simulink model "HEVarchieve"  (R2015a)
settings: Solver=ode45  StartTime=0.0  StopTime=10.0  RelTol=1e-3
undefined symbols (not defined in the file): Hydride, magnitude, Metal, Nickel, Ts
libraries: powerlib x46, driveline x28, simulink_extras x8, electricdrivelib x3, simulink x2, powerlib_extras x2, DC6DriveInternalModels x1
(part 1 of 2)
settings Model: Creator=Elena  LastModifiedBy=Elena

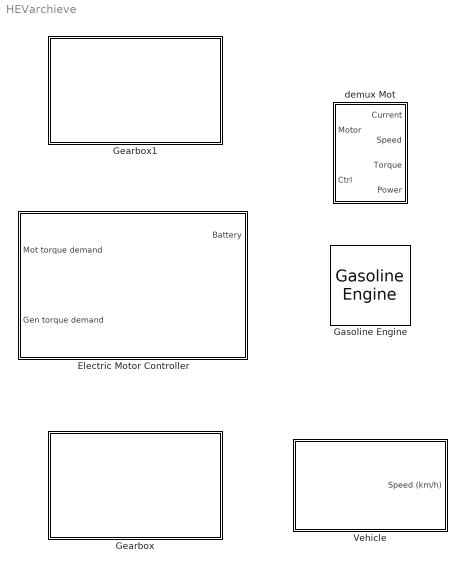
== system HEVarchieve ==
  "Electric Motor Controller " : Subsystem
  Gasoline Engine : driveline/Vehicle Components/Gasoline Engine  power_max=57000  speed_at_power_max=5000  speed_max=6000
      link override Peak torque: LookUpMeth=Interpolation-Extrapolation
  Gearbox : Subsystem
  Gearbox1 : Subsystem
  Vehicle : Subsystem
  demux Mot : Subsystem

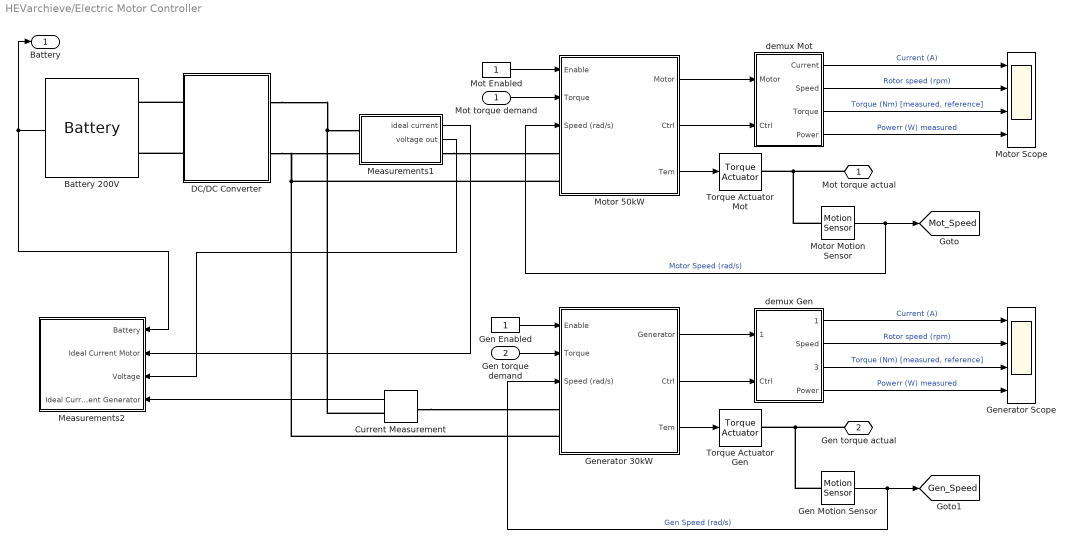
== system HEVarchieve/Electric Motor Controller  ==
  Mot torque demand : Inport
  "Gen torque demand " : Inport  Port=2
  Battery 200V : electricdrivelib/Extra Sources/Battery  BatType=Nickel-Metal-Hydride  ShowDetailedParameters=off  NomV=200  NomQ=6.5  SOC=70  PresetModel=on  MaxQ=7  FullV=235.5932  Dis_rate=1.3  R=0.30769  Normal_OP=6.25  expZone="[216.9492           1.3]"  current=[50 100]  Units=Time  Batt_Tr=30
  Current Measurement : powerlib/Measurements/Current Measurement  PhasorSimulation=off  OutputType=Complex  PSBequivalent=0
  DC/DC Converter : Subsystem
      mask init:
      | [X1,X1m,X2,X2m,X3,X4,Y1,Y1m,Y2,Y2m,Y3,Y4,color1,color2]=spsdrivelogo;
  Gen Enabled : Constant
  Gen Motion Sensor : driveline/Sensors & Actuators/Motion Sensor  Angle=off  x0=0  Velocity=on  Acceleration=off
  Generator 30kW : Subsystem
  Generator Scope : Scope  NumInputPorts=4
      settings: YMin=-5~-5~-5~-5  YMax=5~5~5~5
  Measurements1 : Subsystem
  Measurements2 : Subsystem
  Mot Enabled : Constant
  Motor 50kW : Subsystem
  Motor Motion Sensor : driveline/Sensors & Actuators/Motion Sensor  Angle=off  x0=0  Velocity=on  Acceleration=off
  Motor Scope : Scope  NumInputPorts=4
      settings: YMin=0~0~-100~-5  YMax=250~6000~400~5
  Torque Actuator Gen : driveline/Sensors & Actuators/Torque Actuator
  Torque Actuator Mot : driveline/Sensors & Actuators/Torque Actuator
  demux Gen : Subsystem
  demux Mot : Subsystem
  Mot torque actual : PMIOPort  Port=1  Side=Right
  Gen torque actual : PMIOPort  Port=2  Side=Right
  Battery : Outport
  tag scope: Gen_Speed=global, Mot_Speed=global
  wires:
  Battery 200V/1 -> Measurements2/1(Battery), Battery/1
  Mot Enabled/1 -> Motor 50kW/1(Enable)
  Mot torque demand/1 -> Motor 50kW/2(Torque)
  Motor Motion Sensor/1 -> [Mot_Speed], Motor 50kW/3(Speed (rad/s))  "Motor Speed (rad/s)"
  "Gen torque demand "/1 -> Generator 30kW/2(Torque)
  Gen Enabled/1 -> Generator 30kW/1(Enable)
  Motor 50kW/1(Motor) -> demux Mot/1(Motor)
  Motor 50kW/2(Ctrl) -> demux Mot/2(Ctrl)
  Motor 50kW/3(Tem) -> Torque Actuator Mot/1
  Generator 30kW/3(Tem) -> Torque Actuator Gen/1
  demux Mot/1(Current) -> Motor Scope/1  "Current (A)"
  demux Mot/2(Speed) -> Motor Scope/2  "Rotor speed (rpm)"
  demux Mot/3(Torque) -> Motor Scope/3  "Torque (Nm) [measured, reference]"
  demux Mot/4(Power) -> Motor Scope/4  "Powerr (W) measured"
  Generator 30kW/2(Ctrl) -> demux Gen/2(Ctrl)
  Generator 30kW/1(Generator) -> demux Gen/1(Generator)
  demux Gen/1(Current) -> Generator Scope/1  "Current (A)"
  demux Gen/2(Speed) -> Generator Scope/2  "Rotor speed (rpm)"
  demux Gen/3(Torque) -> Generator Scope/3  "Torque (Nm) [measured, reference]"
  demux Gen/4(Power) -> Generator Scope/4  "Powerr (W) measured"
  Measurements1/2(voltage out) -> Measurements2/3(Voltage)
  Measurements1/1(" ideal current ") -> Measurements2/2(Ideal Current Motor)
  Current Measurement/1 -> Measurements2/4(Ideal Current Generator)
  Gen Motion Sensor/1 -> Generator 30kW/3(Speed (rad/s)), [Gen_Speed]  "Gen Speed (rad/s)"
  connections:
  DC/DC Converter/LConn1 -- Battery 200V/LConn1
  DC/DC Converter/LConn2 -- Battery 200V/LConn2
  Generator 30kW/LConn2 -- Motor 50kW/LConn2 -- Measurements1/LConn2 -- DC/DC Converter/RConn2
  Current Measurement/RConn1 -- DC/DC Converter/RConn1 -- Measurements1/LConn1
  Measurements1/RConn1 -- Motor 50kW/LConn1
  Current Measurement/LConn1 -- Generator 30kW/LConn1
  Gen torque actual/RConn1 -- Torque Actuator Gen/RConn1 -- Gen Motion Sensor/LConn1
  Mot torque actual/RConn1 -- Motor Motion Sensor/LConn1 -- Torque Actuator Mot/RConn1

== system HEVarchieve/Gearbox ==
  Eng Motion Sensor : driveline/Sensors & Actuators/Motion Sensor  Angle=off  x0=0  Velocity=on  Acceleration=off
  Gen Motion Sensor : driveline/Sensors & Actuators/Motion Sensor  Angle=off  x0=0  Velocity=on  Acceleration=off
  Mot Motion Sensor : driveline/Sensors & Actuators/Motion Sensor  Angle=off  x0=0  Velocity=on  Acceleration=off
  Planetary Gear : driveline/Gears/Planetary Gear  Ratio=2.6  Show=off  LinearizationFlag=off  ValidatorFcn=drive_planetarygearblock
  Speed : Scope  NumInputPorts=3
      settings: TimeRange=10  YMin=3.91275~0~37.3  YMax=3.91275~150~37.6  SaveName=ScopeData3  Decimation=10
  T1 : driveline/Sensors & Actuators/Torque Sensor
  Torque Sensor : driveline/Sensors & Actuators/Torque Sensor
  Torque Sensor1 : driveline/Sensors & Actuators/Torque Sensor
  Engine Torque : PMIOPort  Port=1  Side=Left
  Motor Torque : PMIOPort  Port=2  Side=Right
  Generator Torque : PMIOPort  Port=3  Side=Right
  wires:
  Eng Motion Sensor/1 -> Speed/3  "Engine speed (rad/s)"
  Gen Motion Sensor/1 -> Speed/2  "Generator speed (rad/s)"
  Mot Motion Sensor/1 -> Speed/1  "Motor speed (rad/s)"
  connections:
  Torque Sensor/LConn1 -- Planetary Gear/RConn1
  Eng Motion Sensor/LConn1 -- Planetary Gear/LConn1 -- T1/RConn1
  T1/LConn1 -- Engine Torque/RConn1
  Torque Sensor/RConn1 -- Motor Torque/RConn1 -- Mot Motion Sensor/LConn1
  Torque Sensor1/RConn1 -- Gen Motion Sensor/LConn1 -- Generator Torque/RConn1
  Torque Sensor1/LConn1 -- Planetary Gear/RConn2

== system HEVarchieve/Gearbox1 ==
  Eng Motion Sensor : driveline/Sensors & Actuators/Motion Sensor  Angle=off  x0=0  Velocity=on  Acceleration=off
  Gen Motion Sensor : driveline/Sensors & Actuators/Motion Sensor  Angle=off  x0=0  Velocity=on  Acceleration=off
  Mot Motion Sensor : driveline/Sensors & Actuators/Motion Sensor  Angle=off  x0=0  Velocity=on  Acceleration=off
  Planetary Gear : driveline/Gears/Planetary Gear  Ratio=2  Show=off  LinearizationFlag=off  ValidatorFcn=drive_planetarygearblock
  Speed : Scope  NumInputPorts=3
      settings: TimeRange=16  YMin=-100~-20~-200  YMax=500~120~1200  SaveName=ScopeData3  Decimation=10
  Torque Sensor : driveline/Sensors & Actuators/Torque Sensor
  Engine Torque : PMIOPort  Port=1  Side=Left
  Motor Torque : PMIOPort  Port=2  Side=Right
  Generator Torque : PMIOPort  Port=3  Side=Right
  wires:
  Eng Motion Sensor/1 -> Speed/3  "Engine speed (rad/s)"
  Gen Motion Sensor/1 -> Speed/2  "Generator speed (rad/s)"
  Mot Motion Sensor/1 -> Speed/1  "Motor speed (rad/s)"
  connections:
  Planetary Gear/RConn2 -- Gen Motion Sensor/LConn1 -- Generator Torque/RConn1
  Mot Motion Sensor/LConn1 -- Torque Sensor/LConn1 -- Planetary Gear/RConn1 -- Motor Torque/RConn1
  Planetary Gear/LConn1 -- Eng Motion Sensor/LConn1 -- Engine Torque/RConn1

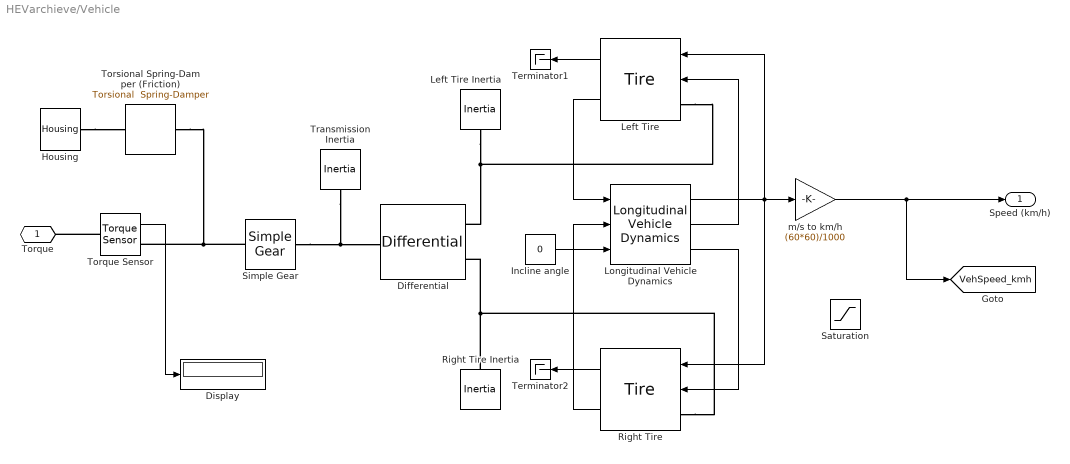
== system HEVarchieve/Vehicle ==
  Differential : driveline/Gears/Differential  R=1  ValidatorFcn=drive_differentialgearblock  SimDrivelineLibraryVersion=1.1
  Display : Display
  Housing : driveline/Solver & Inertias/Housing
  Incline angle : Constant  Value=0
  Left Tire : driveline/Vehicle Components/Tire  r_e=0.3  F_z=3000  F_x_max=3500  kappa_max=10  sigma_k=0.2
  Left Tire Inertia : driveline/Solver & Inertias/Inertia  PortType=p1  BlockClass=Inertia  PhysicalDomain=driveline_domain  I=0.5  Ip=[]  Iv=[]  ShowLeft=off  ShowRight=on
  Longitudinal Vehicle Dynamics : driveline/Vehicle Components/Longitudinal Vehicle Dynamics  m=1325  a=1.35  b=1.35  h=0.5  FA=2.57  C_d=0.26  v0=0
  Right Tire : driveline/Vehicle Components/Tire  r_e=0.3  F_z=3000  F_x_max=3500  kappa_max=10  sigma_k=0.2
  Right Tire Inertia : driveline/Solver & Inertias/Inertia  PortType=p1  BlockClass=Inertia  PhysicalDomain=driveline_domain  I=0.5  Ip=[]  Iv=[]  ShowLeft=off  ShowRight=on
  Saturation : Saturate  UpperLimit=Inf  LowerLimit=0
  Simple Gear : driveline/Gears/Simple Gear  PortType=p1  BlockClass=SimpleGear  PhysicalDomain=driveline_domain  Reversing=off  Ratio=4.113
  Terminator1 : Terminator
  Terminator2 : Terminator
  Torque Sensor : driveline/Sensors & Actuators/Torque Sensor
  Torsional Spring-Damper (Friction) : driveline/Dynamic Elements/Torsional  Spring-Damper  k=0  c=0.1  x0=0  Backlash=0
  Transmission Inertia : driveline/Solver & Inertias/Inertia  PortType=p1  BlockClass=Inertia  PhysicalDomain=driveline_domain  I=0.5  Ip=[]  Iv=[]  ShowLeft=off  ShowRight=on
  m/s to km/h : Gain  Gain=(60*60)/1000
  Torque : PMIOPort  Port=1  Side=Left
  Speed (km/h) : Outport
  tag scope: VehSpeed_kmh=global
  wires:
  Left Tire/2 -> Longitudinal Vehicle Dynamics/1
  Right Tire/2 -> Longitudinal Vehicle Dynamics/2
  Incline angle/1 -> Longitudinal Vehicle Dynamics/3
  Longitudinal Vehicle Dynamics/3 -> Right Tire/2
  Longitudinal Vehicle Dynamics/2 -> Left Tire/2
  Longitudinal Vehicle Dynamics/1 -> m/s to km/h/1, Right Tire/1, Left Tire/1
  Left Tire/1 -> Terminator1/1
  Right Tire/1 -> Terminator2/1
  Torque Sensor/1 -> Display/1
  ? -> Saturation/1
  m/s to km/h/1 -> [VehSpeed_kmh], Speed (km/h)/1
  connections:
  Torque Sensor/LConn1 -- Torque/RConn1
  Torsional Spring-Damper (Friction)/RConn1 -- Simple Gear/LConn1 -- Torque Sensor/RConn1
  Housing/RConn1 -- Torsional Spring-Damper (Friction)/LConn1
  Simple Gear/RConn1 -- Transmission Inertia/RConn1 -- Differential/LConn1
  Left Tire Inertia/RConn1 -- Left Tire/LConn1 -- Differential/RConn1
  Right Tire Inertia/RConn1 -- Right Tire/LConn1 -- Differential/RConn2

== system HEVarchieve/demux Mot ==
  Motor : Inport
  Ctrl : Inport  Port=2
  "+ -> -1" : Gain  Gain=30/pi
  Bus Selector : BusSelector  OutputSignals=Stator current is_a (A),Rotor speed wm (rad/s),Electromagnetic torque Te (N*m)
  Bus Selector1 : BusSelector  OutputSignals=Torque reference (Nm)
  Mux1 : Mux  Inputs=2
  Product : Product  RndMeth=Zero
  Current : Outport
  Speed : Outport  Port=2
  Torque : Outport  Port=3
  Power : Outport  Port=4
  wires:
  "+ -> -1"/1 -> Speed/1
  Motor/1 -> Bus Selector/1
  Ctrl/1 -> Bus Selector1/1
  Bus Selector/2 -> "+ -> -1"/1, Product/2  "<Rotor speed wm (rad/s)>"
  Bus Selector/3 -> Product/1, Mux1/1  "<Electromagnetic torque Te (N*m)>"
  Bus Selector1/1 -> Mux1/2  "<Torque reference (Nm)>"
  Mux1/1 -> Torque/1
  Bus Selector/1 -> Current/1  "<Stator current is_a (A)>"
  Product/1 -> Power/1

== system HEVarchieve/Electric Motor Controller /DC//DC Converter ==
  Bus DC controller : Subsystem
  DC/DC converter : Subsystem
  Ubus Ref : Constant  Value=500
  +VDC : PMIOPort  Tag=PMCPort  Port=1  Side=Right
  -VDC : PMIOPort  Tag=PMCPort  Port=2  Side=Right
  + Bat : PMIOPort  Tag=PMCPort  Port=3  Side=Left
  - Bat : PMIOPort  Tag=PMCPort  Port=4  Side=Left
  wires:
  Ubus Ref/1 -> Bus DC controller/2(Uref)
  Bus DC controller/1(Duty cycle) -> DC/DC converter/1(Duty Cycle)
  DC/DC converter/1(UBus) -> Bus DC controller/1(Ubus)
  connections:
  +VDC/RConn1 -- DC/DC converter/LConn1
  -VDC/RConn1 -- DC/DC converter/LConn2
  + Bat/RConn1 -- DC/DC converter/RConn1
  - Bat/RConn1 -- DC/DC converter/RConn2

== system HEVarchieve/Electric Motor Controller /Generator 30kW ==
  Enable : Inport
  Torque : Inport  Port=2
  Speed (rad/s) : Inport  Port=3
  Bus Selector : BusSelector  OutputSignals=Rotor speed wm (rad/s),Rotor angle thetam (rad),Electromagnetic torque Te (N*m)
  Measures : electricdrivelib/AC drives/PM Synchronous Motor Drive/Measures
  Mux : Subsystem
  PMSM1 : powerlib/Machines/Permanent Magnet Synchronous Machine  NbPhases=3  FluxDistribution=Sinusoidal  RotorType=Salient-pole  MechanicalLoad=Speed w  PresetModel=No  ShowDetailedParameters=on  MeasurementBus=off  Resistance=0.05  Inductance=0  dqInductances=[0.000635 0.000635]  La=0.000835  MachineConstant=Flux linkage established by magnets (V.s)  Flux=0.192  VoltageCst=34.8249  TorqueCst=0.288  Flat=0  Mechanical=[0.011 0.001889/4 4/4]  PolePairs=1  InitialConditions=[0,0, 0,0,0]  InitialConditions5ph=[0 0 0 0 0 0]  TsPowergui=0  TsBlock=-1  RefAngle=90 degrees behind phase A axis (modified Park)
      settings: AttributesFormatString=\n
  Speed Controller : Subsystem  mask(Speed controller){SwK=Torque regulation, bs=1800, ramp=[-5000,5000], kp=(1/5)/4, ki=(50/5)/4/3, fc=(1000/10)/2, ctrl_sat=[-45,45], Tsc=Ts}
      mask prompts: SwK "Regulation type"; bs "Base speed (rpm)"; ramp "Speed reference ramp (rpm/s) [deceleration,acceleration]"; kp "Proportional gain"; ki "Integral gain"; fc "Speed measurement - low-pass filter cutoff frequency (Hz)"; ctrl_sat "Controller output torque saturation (N.m) [negative,positive]"; Tsc "Controller sampling time (s)"
      mask help: This block implements a PI speed regulator.
      mask init:
      | [X1,X1m,X2,X2m,X3,X4,Y1,Y1m,Y2,Y2m,Y3,Y4,color1,color2]=spsdrivelogo;
      mask TypeOptions SwK: Speed regulation | Torque regulation
      mask Display:
      | patch([X1 X1m],[Y1 Y1m],color1);
      | patch(X3,Y3,color2);
      | plot([X1 X1m X2 X2m X3 X4],[Y1 Y1m Y2 Y2m Y3 Y4]);
  Three-phase Inverter : Subsystem  mask(SPSdrives Converter){Arms=3, SnubberResistance=5000, SnubberCapacitance=inf, Device=IGBT / Diodes, Ron=1e-3, Lon=0, ForwardVoltages=[0.8,0.8], ForwardVoltage=0, GTOparameters=[0,0], IGBTparameters=[1e-6,2e-6], Measurements=All voltages and currents, SourceFrequency=60, dqInductances=[0.000635,0.000635], Flux=0.192, Resistance=0.05, p=4/4, converterType=Inverter}
      mask prompts: Arms "Number of bridge arms:"; SnubberResistance "Snubber resistance Rs (Ohms)"; SnubberCapacitance "Snubber capacitance Cs (F)"; Device "Power Electronic device"; Ron "Ron (Ohms)"; Lon "Lon (H)"; ForwardVoltages "Forward voltages  [ Device Vf(V) , Diode Vfd(V)]"; ForwardVoltage "Forward voltage Vf (V)"; GTOparameters "[  Tf (s) , Tt (s)  ]"; IGBTparameters "[  Tf (s) , Tt (s)  ]"; SourceFrequency "Source Frequency (Hz)"; dqInductances "PMSM-Inductances [ Ld(H) Lq(H) ]:"; Flux "PMSM-Flux induced by magnets (Wb):"; Resistance "PMSM-Stator resistance Rs (ohm):"; p "PMSM-Pairs of poles p:"; converterType "Converter type:"
      mask init:
      | Ld=dqInductances(1);
      | Lq=dqInductances(2);
      | Fcs=6*SourceFrequency/10;
      settings: OpenFcn=power_openblockproxy();
      mask Help: web(psbhelp);
      mask TypeOptions Arms: 1 | 2 | 3
      mask TypeOptions Device: Diodes | Thyristors | GTO / Diodes | MOSFET / Diodes | IGBT / Diodes | Ideal Switches
      mask TypeOptions Measurements: None | Device voltages | Device currents | UAB UBC UCA UDC voltages | All voltages and currents
      mask TypeOptions converterType: Rectifier | Inverter
      mask Display: plot(0,0,100,100,[39 39 23.8],[71 28 28],[44 56 49.6 56 52.8 56 61 61],[39.2 33.6 32.8 33.6 40.8 33.6 30 12.4],[44 44 44 61 61],[28 71 60 66.4 90],[75 67 83 75 67 83 75 75],[54 42 42 54 54 54 54 66],[61 75 75],[24 24 42],[75 75 61],[66,76,76])
  VECT : Subsystem  mask(VECT){nb_p=4/4, lambda=0.192, freq_max=20e3, Ts_vect=Ts, h=2}
      mask prompts: nb_p "Motor pairs of poles"; lambda "Flux induced by magnets (Wb)"; freq_max "Maximum switching frequency (Hz)"; Ts_vect "Sampling time (s)"; h "Current hysteresis bandwidth (A)"
      mask help: This block implements a vector controller.
      mask init:
      | [X1,X1m,X2,X2m,X3,X4,Y1,Y1m,Y2,Y2m,Y3,Y4,color1,color2]=spsdrivelogo;
      mask Display:
      | patch([X1 X1m],[Y1 Y1m],color1);
      | patch(X3,Y3,color2);
      | plot([X1 X1m X2 X2m X3 X4],[Y1 Y1m Y2 Y2m Y3 Y4]);
  + : PMIOPort  Port=1  Side=Left
  - : PMIOPort  Port=2  Side=Left
  Generator : Outport
  Ctrl : Outport  Port=2
  Tem : Outport  Port=3
  wires:
  Enable/1 -> VECT/1(En), Speed Controller/3(En)
  Torque/1 -> Speed Controller/2(N*)
  Speed Controller/1(Torque*) -> VECT/2(Torque*)
  Bus Selector/1 -> Speed Controller/1(N)  "<Rotor speed wm (rad/s)>"
  PMSM1/1 -> Mux/2(m), Bus Selector/1, Generator/1
  Speed (rad/s)/1 -> PMSM1/1
  Bus Selector/3 -> Tem/1  "<Electromagnetic torque Te (N*m)>"
  Measures/1 -> VECT/4(I_abc)
  Speed Controller/2(Ctrl) -> Ctrl/1
  VECT/1(sig*) -> Mux/1(sig*)
  Mux/1(Ctrl) -> Three-phase Inverter/1(ctrl)
  Bus Selector/2 -> VECT/3(teta)  "<Rotor angle thetam (rad)>"
  connections:
  -/RConn1 -- Three-phase Inverter/RConn2
  +/RConn1 -- Three-phase Inverter/RConn1
  Measures/RConn1 -- PMSM1/LConn1
  Measures/RConn2 -- PMSM1/LConn2
  Measures/RConn3 -- PMSM1/LConn3
  Three-phase Inverter/LConn1 -- Measures/LConn1
  Measures/LConn2 -- Three-phase Inverter/LConn2
  Three-phase Inverter/LConn3 -- Measures/LConn3

== system HEVarchieve/Electric Motor Controller /Measurements1 ==
  Current : powerlib/Measurements/Current Measurement  PhasorSimulation=off  OutputType=Complex  PSBequivalent=0
  Voltage : powerlib/Measurements/Voltage Measurement  PhasorSimulation=off  OutputType=Complex  PSBequivalent=0
  ideal current ref : PMIOPort  Port=1  Side=Right
  + : PMIOPort  Tag=PMCPort  Port=2  Side=Left
  - : PMIOPort  Port=3  Side=Left
  " ideal current " : Outport
  voltage out : Outport  Port=2
  wires:
  Voltage/1 -> voltage out/1
  Current/1 -> " ideal current "/1
  connections:
  -/RConn1 -- Voltage/LConn2
  ideal current ref/RConn1 -- Current/RConn1
  Current/LConn1 -- Voltage/LConn1 -- +/RConn1

== system HEVarchieve/Electric Motor Controller /Measurements2 ==
  Battery : Inport
  Ideal Current Motor : Inport  Port=2
  Voltage : Inport  Port=3
  Ideal Current Generator : Inport  Port=4
  Bus Selector1 : BusSelector  OutputSignals=SOC (%),Current (A),Voltage (V)
  Mux3 : Mux  Inputs=3
  Mux4 : Mux  Inputs=3
  Mux5 : Mux  Inputs=2
  Product1 : Product  RndMeth=Zero
  Product2 : Product  RndMeth=Zero
  Product3 : Product  RndMeth=Zero
  Scope : Scope  NumInputPorts=3
      settings: YMin=-1.38778e-17~200~66.4999  YMax=0.2~500~73.4999  SaveName=ScopeData2
  tag scope: Power=global
  wires:
  Battery/1 -> Bus Selector1/1
  Bus Selector1/1 -> Scope/3  "<SOC (%)>"
  Bus Selector1/2 -> Product3/1, Mux4/3  "<Current (A)>"
  Bus Selector1/3 -> Mux5/2, Product3/2  "<Voltage (V)>"
  Product3/1 -> Mux3/3  "Battery Power (W)"
  Ideal Current Motor/1 -> Mux4/1, Product1/1
  Voltage/1 -> Product1/2, Product2/2, Mux5/1
  Product1/1 -> Mux3/1  "Motor Power (W)"
  Ideal Current Generator/1 -> Mux4/2, Product2/1
  Product2/1 -> Mux3/2  "Generator Power (W)"
  Mux4/1 -> Scope/1  "Current (Motor + Generator + Battery)"
  Mux5/1 -> Scope/2  "Voltage ( DC Bus + Battery)"
  Mux3/1 -> [Power]

== system HEVarchieve/Electric Motor Controller /Motor 50kW ==
  Enable : Inport
  Torque : Inport  Port=2
  Speed (rad/s) : Inport  Port=3
  500 VDC 50kW PMSM : powerlib/Machines/Permanent Magnet Synchronous Machine  NbPhases=3  FluxDistribution=Sinusoidal  RotorType=Salient-pole  MechanicalLoad=Speed w  PresetModel=No  ShowDetailedParameters=on  MeasurementBus=off  Resistance=0.0065  Inductance=0  dqInductances="[0.001597972349731   0.002057052250467]"  La=0.000835  MachineConstant=Flux linkage established by magnets (V.s)  Flux=0.175666143629361  VoltageCst=127.4493  TorqueCst=1.054  Flat=0  Mechanical=[0.089 0.005 4]  PolePairs=4  InitialConditions=[0,0,0,0]  InitialConditions5ph=[0 0 0 0 0 0]  TsPowergui=0  TsBlock=-1  RefAngle=90 degrees behind phase A axis (modified Park)
      settings: AttributesFormatString=\n
  Bus Selector : BusSelector  OutputSignals=Rotor speed wm (rad/s),Rotor angle thetam (rad),Electromagnetic torque Te (N*m)
  Measures : electricdrivelib/AC drives/PM Synchronous Motor Drive/Measures
  Mux : Subsystem
  Speed Controller : Subsystem  mask(Speed controller){SwK=Torque regulation, bs=3000, ramp=[-10000,10000], kp=1/5, ki=50/5, fc=1000/10, ctrl_sat=[-400,400], Tsc=Ts}
      mask prompts: SwK "Regulation type"; bs "Base speed (rpm)"; ramp "Speed reference ramp (rpm/s) [deceleration,acceleration]"; kp "Proportional gain"; ki "Integral gain"; fc "Speed measurement - low-pass filter cutoff frequency (Hz)"; ctrl_sat "Controller output torque saturation (N.m) [negative,positive]"; Tsc "Controller sampling time (s)"
      mask help: This block implements a PI speed regulator.
      mask init:
      | [X1,X1m,X2,X2m,X3,X4,Y1,Y1m,Y2,Y2m,Y3,Y4,color1,color2]=spsdrivelogo;
      mask TypeOptions SwK: Speed regulation | Torque regulation
      mask Display:
      | patch([X1 X1m],[Y1 Y1m],color1);
      | patch(X3,Y3,color2);
      | plot([X1 X1m X2 X2m X3 X4],[Y1 Y1m Y2 Y2m Y3 Y4]);
  Three-phase Inverter : Subsystem  mask(SPSdrives Converter){Arms=3, SnubberResistance=5000, SnubberCapacitance=inf, Device=IGBT / Diodes, Ron=1e-3, Lon=0, ForwardVoltages=[0.8,0.8], ForwardVoltage=0, GTOparameters=[0,0], IGBTparameters=[1e-6,2e-6], Measurements=All voltages and currents, SourceFrequency=60, dqInductances=[0.001597972349731   0.002057052250467], Flux=0.175666143629361, Resistance=0.0065, p=4, converterType=Inverter}
      mask prompts: Arms "Number of bridge arms:"; SnubberResistance "Snubber resistance Rs (Ohms)"; SnubberCapacitance "Snubber capacitance Cs (F)"; Device "Power Electronic device"; Ron "Ron (Ohms)"; Lon "Lon (H)"; ForwardVoltages "Forward voltages  [ Device Vf(V) , Diode Vfd(V)]"; ForwardVoltage "Forward voltage Vf (V)"; GTOparameters "[  Tf (s) , Tt (s)  ]"; IGBTparameters "[  Tf (s) , Tt (s)  ]"; SourceFrequency "Source Frequency (Hz)"; dqInductances "PMSM-Inductances [ Ld(H) Lq(H) ]:"; Flux "PMSM-Flux induced by magnets (Wb):"; Resistance "PMSM-Stator resistance Rs (ohm):"; p "PMSM-Pairs of poles p:"; converterType "Converter type:"
      mask init:
      | Ld=dqInductances(1);
      | Lq=dqInductances(2);
      | Fcs=6*SourceFrequency/10;
      settings: OpenFcn=power_openblockproxy();
      mask Help: web(psbhelp);
      mask TypeOptions Arms: 1 | 2 | 3
      mask TypeOptions Device: Diodes | Thyristors | GTO / Diodes | MOSFET / Diodes | IGBT / Diodes | Ideal Switches
      mask TypeOptions Measurements: None | Device voltages | Device currents | UAB UBC UCA UDC voltages | All voltages and currents
      mask TypeOptions converterType: Rectifier | Inverter
      mask Display: plot(0,0,100,100,[39 39 23.8],[71 28 28],[44 56 49.6 56 52.8 56 61 61],[39.2 33.6 32.8 33.6 40.8 33.6 30 12.4],[44 44 44 61 61],[28 71 60 66.4 90],[75 67 83 75 67 83 75 75],[54 42 42 54 54 54 54 66],[61 75 75],[24 24 42],[75 75 61],[66,76,76])
  Torque limitation : Subsystem
      mask Display: plot([0;1800;2000;2500;3000;3500], [1;1;0.90*1;0.72*1;0.6*1;0.51*1])
  VECT controller : Subsystem  mask(VECT){nb_p=4, dqInductances=[0.001597972349731   0.002057052250467], lambda=0.175666143629361, Ts_vect=60e-6}
      mask prompts: nb_p "Motor pairs of poles"; dqInductances "Inductances [ Ld(H) Lq(H) ]:"; lambda "Flux induced by magnets (Wb)"; Ts_vect "Sampling time (s)"
      mask help: This block implements a vector controller.
      mask init:
      | [X1,X1m,X2,X2m,X3,X4,Y1,Y1m,Y2,Y2m,Y3,Y4,color1,color2]=spsdrivelogo;
      | ib = lambda/(dqInductances(2)-dqInductances(1));
      | Teb = 3/2*nb_p*lambda*ib;
      | Ld = dqInductances(1);
      | Lq = dqInductances(2);
      | lam = lambda;
      | p=nb_p;
      | ib = lam/(Lq-Ld);
      | iqn = 0:0.01:3;
      | ten = iqn/2.*(sqrt(4*iqn.*iqn+1)+1);
      mask Display:
      | patch([X1 X1m],[Y1 Y1m],color1);
      | patch(X3,Y3,color2);
      | plot([X1 X1m X2 X2m X3 X4],[Y1 Y1m Y2 Y2m Y3 Y4]);
  + : PMIOPort  Port=1  Side=Left
  - : PMIOPort  Port=2  Side=Left
  Motor : Outport
  Ctrl : Outport  Port=2
  Tem : Outport  Port=3
  wires:
  Mux/1(Ctrl) -> Three-phase Inverter/1(ctrl)
  VECT controller/1(sig*) -> Mux/1(sig)
  Speed Controller/2(Ctrl) -> Ctrl/1
  Speed (rad/s)/1 -> 500 VDC 50kW PMSM/1
  500 VDC 50kW PMSM/1 -> Bus Selector/1, Mux/2(m), Motor/1
  Bus Selector/3 -> Tem/1  "<Electromagnetic torque Te (N*m)>"
  Bus Selector/1 -> VECT controller/3(w), Speed Controller/1(N), Torque limitation/1(N rad/s)  "<Rotor speed wm (rad/s)>"
  Enable/1 -> VECT controller/1(En), Speed Controller/3(En)
  Speed Controller/1(Torque*) -> VECT controller/2(Torque*)
  Measures/1 -> VECT controller/5(I_abc)
  Bus Selector/2 -> VECT controller/4(teta)  "<Rotor angle thetam (rad)>"
  Torque limitation/1(torque) -> Speed Controller/2(N*)
  Torque/1 -> Torque limitation/2(Torque)
  connections:
  Three-phase Inverter/LConn3 -- Measures/LConn3
  Measures/LConn2 -- Three-phase Inverter/LConn2
  Three-phase Inverter/LConn1 -- Measures/LConn1
  Measures/RConn3 -- 500 VDC 50kW PMSM/LConn3
  Measures/RConn2 -- 500 VDC 50kW PMSM/LConn2
  Measures/RConn1 -- 500 VDC 50kW PMSM/LConn1
  +/RConn1 -- Three-phase Inverter/RConn1
  -/RConn1 -- Three-phase Inverter/RConn2

== system HEVarchieve/Electric Motor Controller /demux Gen ==
  Generator : Inport
  Ctrl : Inport  Port=2
  "+ -> -1" : Gain  Gain=30/pi
  Bus Selector : BusSelector  OutputSignals=Stator current is_a (A),Rotor speed wm (rad/s),Electromagnetic torque Te (N*m)
  Bus Selector1 : BusSelector  OutputSignals=Torque reference (Nm)
  Mux1 : Mux  Inputs=2
  Product : Product  RndMeth=Zero
  Current : Outport
  Speed : Outport  Port=2
  Torque : Outport  Port=3
  Power : Outport  Port=4
  wires:
  "+ -> -1"/1 -> Speed/1
  Generator/1 -> Bus Selector/1
  Ctrl/1 -> Bus Selector1/1
  Bus Selector/2 -> Product/2, "+ -> -1"/1  "<Rotor speed wm (rad/s)>"
  Bus Selector/3 -> Product/1, Mux1/1  "<Electromagnetic torque Te (N*m)>"
  Bus Selector1/1 -> Mux1/2  "<Torque reference (Nm)>"
  Mux1/1 -> Torque/1
  Bus Selector/1 -> Current/1  "<Stator current is_a (A)>"
  Product/1 -> Power/1

== system HEVarchieve/Electric Motor Controller /demux Mot ==
  Motor : Inport
  Ctrl : Inport  Port=2
  "+ -> -1" : Gain  Gain=30/pi
  Bus Selector : BusSelector  OutputSignals=Stator current is_a (A),Rotor speed wm (rad/s),Electromagnetic torque Te (N*m)
  Bus Selector1 : BusSelector  OutputSignals=Torque reference (Nm)
  Mux1 : Mux  Inputs=2
  Product : Product  RndMeth=Zero
  Current : Outport
  Speed : Outport  Port=2
  Torque : Outport  Port=3
  Power : Outport  Port=4
  wires:
  "+ -> -1"/1 -> Speed/1
  Motor/1 -> Bus Selector/1
  Ctrl/1 -> Bus Selector1/1
  Bus Selector/2 -> "+ -> -1"/1, Product/2  "<Rotor speed wm (rad/s)>"
  Bus Selector/3 -> Product/1, Mux1/1  "<Electromagnetic torque Te (N*m)>"
  Bus Selector1/1 -> Mux1/2  "<Torque reference (Nm)>"
  Mux1/1 -> Torque/1
  Bus Selector/1 -> Current/1  "<Stator current is_a (A)>"
  Product/1 -> Power/1

== system HEVarchieve/Electric Motor Controller /DC//DC Converter/Bus DC controller ==
  Ubus : Inport
  Uref : Inport  Port=2
  Current controller DISCRETE1 : Subsystem  mask(PI controller){Kp=0.001, Ki=1, Ts=Ts}
      mask prompts: Kp "Proportional gain (Kp)"; Ki "Integral gain (Ki)"; Ts "Sample time (s) :"
      mask help: Proportional-Integral Speed Controller
      mask Display: plot(0,0,100,100,[35,35,65],[70,30,30],[35,65],[45,60])
  Duty Cycles : Subsystem
  Mux : Mux  Inputs=2
  Transfer Fcn : TransferFcn  Denominator=[.0001 1]
  Unit Delay2 : UnitDelay  InitialCondition=.5  SampleTime=Ts
  Zero-Order Hold1 : ZeroOrderHold  SampleTime=Ts
  Duty cycle : Outport  InitialOutput=0
  tag scope: V_DCDC=global
  wires:
  Ubus/1 -> Zero-Order Hold1/1, Mux/2
  Uref/1 -> Current controller DISCRETE1/2(Uref), Mux/1
  Zero-Order Hold1/1 -> Transfer Fcn/1
  Unit Delay2/1 -> Duty cycle/1
  Transfer Fcn/1 -> Current controller DISCRETE1/1(UBus)
  Current controller DISCRETE1/1(Ec) -> Duty Cycles/1(Ec)
  Duty Cycles/1(dc) -> Unit Delay2/1
  Mux/1 -> [V_DCDC]

== system HEVarchieve/Electric Motor Controller /DC//DC Converter/DC//DC converter ==
  Duty Cycle : Inport
  CBus : powerlib/Elements/Series RLC Branch  LConnTagsString=__new0  RConnTagsString=__new0  BranchType=RC  Resistance=0.2  Inductance=1e-3  SetiL0=off  InitialCurrent=0  Capacitance=1130e-6  Setx0=on  InitialVoltage=500  Measurements=None
  CBus1 : powerlib/Elements/Series RLC Branch  LConnTagsString=__new0  RConnTagsString=__new0  BranchType=C  Resistance=0.2  Inductance=1e-3  SetiL0=off  InitialCurrent=0  Capacitance=282e-6  Setx0=on  InitialVoltage=150  Measurements=None
  Chopper : DC6DriveInternalModels/Chopper (average model)  SnubberResistance=10e3  SnubberCapacitance=inf  Ron=1e-3  ForwardVoltages=[1.3,1.3]  IGBTParameters=[0,0]  converterType=Inverter
  L : powerlib/Elements/Series RLC Branch  LConnTagsString=__new0  RConnTagsString=__new0  BranchType=L  Resistance=0.3  Inductance=373e-6  SetiL0=off  InitialCurrent=100  Capacitance=100e-6  Setx0=off  InitialVoltage=0  Measurements=None
  Neutral2 : powerlib/Elements/Neutral  LConnTagsString=a  NodeNumber=10
  V1 : powerlib/Measurements/Voltage Measurement  PhasorSimulation=off  OutputType=Complex  PSBequivalent=0
  + : PMIOPort  Tag=PMCPort  Port=1  Side=Left
  - : PMIOPort  Tag=PMCPort  Port=2  Side=Left
  + bat. : PMIOPort  Tag=PMCPort  Port=3  Side=Right
  - bat. : PMIOPort  Tag=PMCPort  Port=4  Side=Right
  UBus : Outport
  wires:
  Duty Cycle/1 -> Chopper/1
  V1/1 -> UBus/1
  connections:
  Chopper/RConn1 -- L/RConn1
  L/LConn1 -- + bat./RConn1 -- CBus1/LConn1
  CBus1/RConn1 -- - bat./RConn1 -- Chopper/LConn2 -- -/RConn1 -- CBus/RConn1 -- V1/LConn2 -- Neutral2/LConn1
  +/RConn1 -- CBus/LConn1 -- Chopper/LConn1 -- V1/LConn1

== system HEVarchieve/Electric Motor Controller /Generator 30kW/Mux ==
  sig* : Inport
  m : Inport  Port=2
  Bus Creator : BusCreator  Inputs=2
  Ctrl : Outport
  wires:
  m/1 -> Bus Creator/2  "m"
  sig*/1 -> Bus Creator/1  "Signals*"
  Bus Creator/1 -> Ctrl/1

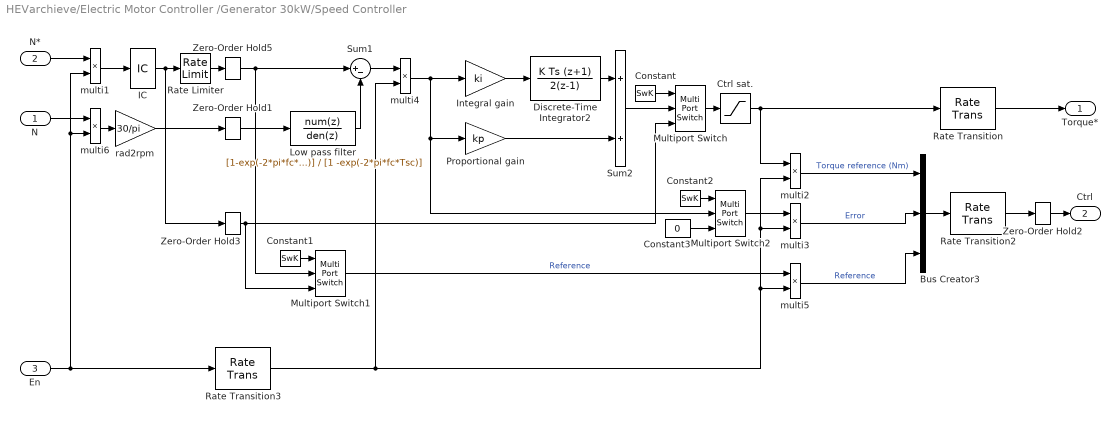
== system HEVarchieve/Electric Motor Controller /Generator 30kW/Speed Controller ==
  N : Inport
  N* : Inport  Port=2
  En : Inport  Port=3
  Bus Creator3 : BusCreator  Inputs=3
  Constant : Constant  Value=SwK
  Constant1 : Constant  Value=SwK
  Constant2 : Constant  Value=SwK
  Constant3 : Constant  Value=0
  Ctrl sat. : Saturate  UpperLimit=ctrl_sat(2)  LowerLimit=ctrl_sat(1)
  Discrete-Time Integrator2 : DiscreteIntegrator  IntegratorMethod=Integration: Trapezoidal  SampleTime=Tsc  LimitOutput=on  UpperSaturationLimit=ctrl_sat(2)  LowerSaturationLimit=ctrl_sat(1)
  IC : InitialCondition  Value=0
  Integral gain : Gain  Gain=ki  SaturateOnIntegerOverflow=on  OutDataTypeStr=Inherit: Same as input  ParamDataTypeStr=Inherit: Same as input
  Low pass filter : DiscreteTransferFcn  Numerator=[1-exp(-2*pi*fc*Tsc)]  Denominator=[1 -exp(-2*pi*fc*Tsc)]  SampleTime=Tsc
  Multiport Switch : MultiPortSwitch  Inputs=2  SaturateOnIntegerOverflow=on
  Multiport Switch1 : MultiPortSwitch  Inputs=2  SaturateOnIntegerOverflow=on
  Multiport Switch2 : MultiPortSwitch  Inputs=2  SaturateOnIntegerOverflow=on
  Proportional gain : Gain  Gain=kp  SaturateOnIntegerOverflow=on  OutDataTypeStr=Inherit: Same as input  ParamDataTypeStr=Inherit: Same as input
  Rate Limiter : RateLimiter  RisingSlewLimit=ramp(2)  FallingSlewLimit=ramp(1)  LinearizeAsGain=off
  Rate Transition : RateTransition
  Rate Transition2 : RateTransition
  Rate Transition3 : RateTransition
  Sum1 : Sum  Inputs=|+-  SaturateOnIntegerOverflow=on  InputSameDT=on  OutDataTypeStr=Inherit: Same as first input
  Sum2 : Sum  SaturateOnIntegerOverflow=on  InputSameDT=on  OutDataTypeStr=Inherit: Same as first input
  Zero-Order Hold1 : ZeroOrderHold  SampleTime=Tsc
  Zero-Order Hold2 : ZeroOrderHold  SampleTime=Ts
  Zero-Order Hold3 : ZeroOrderHold  SampleTime=Tsc
  Zero-Order Hold5 : ZeroOrderHold  SampleTime=Tsc
  multi{1..6} (6 alike) : Product
  rad2rpm : Gain  Gain=30/pi  SaturateOnIntegerOverflow=on  OutDataTypeStr=Inherit: Same as input  ParamDataTypeStr=Inherit: Same as input
  Torque* : Outport
  Ctrl : Outport  Port=2
  wires:
  N/1 -> multi6/1
  multi6/1 -> rad2rpm/1
  N*/1 -> multi1/1
  multi1/1 -> IC/1
  Rate Transition3/1 -> multi5/2, multi2/2, multi3/2, multi4/2
  multi4/1 -> Multiport Switch2/2, Proportional gain/1, Integral gain/1
  Low pass filter/1 -> Sum1/2
  multi2/1 -> Bus Creator3/1  "Torque reference (Nm)"
  Multiport Switch1/1 -> multi5/1  "Reference"
  multi5/1 -> Bus Creator3/3  "Reference"
  multi3/1 -> Bus Creator3/2  "Error"
  Multiport Switch2/1 -> multi3/1
  Zero-Order Hold2/1 -> Ctrl/1
  Rate Transition/1 -> Torque*/1
  En/1 -> multi6/2, multi1/2, Rate Transition3/1
  rad2rpm/1 -> Zero-Order Hold1/1
  Constant3/1 -> Multiport Switch2/3
  Constant2/1 -> Multiport Switch2/1
  Zero-Order Hold3/1 -> Multiport Switch1/3, Multiport Switch/3
  Constant1/1 -> Multiport Switch1/1
  Sum2/1 -> Multiport Switch/2
  Constant/1 -> Multiport Switch/1
  Multiport Switch/1 -> Ctrl sat./1
  Zero-Order Hold5/1 -> Multiport Switch1/2, Sum1/1
  Rate Limiter/1 -> Zero-Order Hold5/1
  Bus Creator3/1 -> Rate Transition2/1
  Rate Transition2/1 -> Zero-Order Hold2/1
  Zero-Order Hold1/1 -> Low pass filter/1
  IC/1 -> Zero-Order Hold3/1, Rate Limiter/1
  Proportional gain/1 -> Sum2/2
  Discrete-Time Integrator2/1 -> Sum2/1
  Sum1/1 -> multi4/1
  Integral gain/1 -> Discrete-Time Integrator2/1
  Ctrl sat./1 -> multi2/1, Rate Transition/1

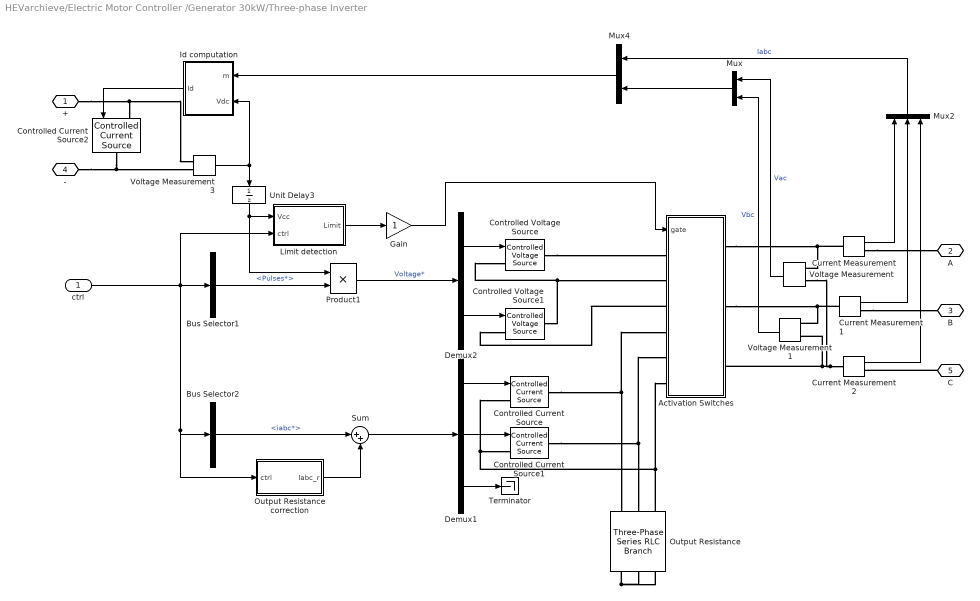
== system HEVarchieve/Electric Motor Controller /Generator 30kW/Three-phase Inverter ==
  ctrl : Inport
  Activation Switches : Subsystem
  Bus Selector1 : BusSelector  OutputSignals=Signals*.Pulses*
  Bus Selector2 : BusSelector  OutputSignals=Signals*.iabc*
  Controlled Current Source : powerlib/Electrical Sources/Controlled Current Source  Initialize=on  Source_Type=AC  Amplitude=0  Phase=0  Frequency=0  Measurements=None
  Controlled Current Source1 : powerlib/Electrical Sources/Controlled Current Source  Initialize=on  Source_Type=AC  Amplitude=0  Phase=0  Frequency=0  Measurements=None
  Controlled Current Source2 : powerlib/Electrical Sources/Controlled Current Source  Initialize=on  Source_Type=AC  Amplitude=0  Phase=0  Frequency=0  Measurements=None
  Controlled Voltage Source : powerlib/Electrical Sources/Controlled Voltage Source  Initialize=on  Source_Type=AC  Amplitude=0  Phase=0  Frequency=0  Measurements=None
  Controlled Voltage Source1 : powerlib/Electrical Sources/Controlled Voltage Source  Initialize=on  Source_Type=AC  Amplitude=0  Phase=0  Frequency=0  Measurements=None
  Current Measurement : powerlib/Measurements/Current Measurement  PhasorSimulation=off  OutputType=Complex  PSBequivalent=0
  Current Measurement1 : powerlib/Measurements/Current Measurement  PhasorSimulation=off  OutputType=Complex  PSBequivalent=0
  Current Measurement2 : powerlib/Measurements/Current Measurement  PhasorSimulation=off  OutputType=Complex  PSBequivalent=0
  Demux1 : Demux  Outputs=3
  Demux2 : Demux  Outputs=2
  Gain : Gain
  Id computation : Subsystem
  Limit detection : Subsystem
  Mux : Mux  Inputs=2
  Mux2 : Mux  Inputs=3
  Mux4 : Mux  Inputs=2
  Output Resistance : powerlib/Elements/Three-Phase Series RLC Branch  LConnTagsString=A|B|C  RConnTagsString=A|B|C  BranchType=R  Resistance=100*Resistance  Inductance=1e-3  Capacitance=1e-6  Measurements=Branch voltages and currents
  Output Resistance correction : Subsystem
  Product1 : Product  RndMeth=Zero
  Sum : Sum  Inputs=|++
  Terminator : Terminator
  Unit Delay3 : UnitDelay  SampleTime=Ts
  Voltage Measurement : powerlib/Measurements/Voltage Measurement  PhasorSimulation=off  OutputType=Complex  PSBequivalent=0
  Voltage Measurement1 : powerlib/Measurements/Voltage Measurement  PhasorSimulation=off  OutputType=Complex  PSBequivalent=0
  Voltage Measurement3 : powerlib/Measurements/Voltage Measurement  PhasorSimulation=off  OutputType=Complex  PSBequivalent=0
  + : PMIOPort  Port=1  Side=Right
  A : PMIOPort  Port=2  Side=Left
  B : PMIOPort  Port=3  Side=Left
  - : PMIOPort  Port=4  Side=Right
  C : PMIOPort  Port=5  Side=Left
  wires:
  Gain/1 -> Activation Switches/1(gate)
  Output Resistance correction/1("Iabc_r ") -> Sum/2
  Product1/1 -> Demux2/1  "Voltage*"
  ctrl/1 -> Output Resistance correction/1(ctrl), Bus Selector2/1, Limit detection/2(ctrl), Bus Selector1/1
  Unit Delay3/1 -> Limit detection/1(Vcc), Product1/1
  Sum/1 -> Demux1/1
  Limit detection/1(Limit) -> Gain/1
  Bus Selector2/1 -> Sum/1  "<iabc*>"
  Demux2/1 -> Controlled Voltage Source/1
  Demux2/2 -> Controlled Voltage Source1/1
  Demux1/3 -> Terminator/1
  Demux1/2 -> Controlled Current Source1/1
  Demux1/1 -> Controlled Current Source/1
  Bus Selector1/1 -> Product1/2  "<Pulses*>"
  Voltage Measurement3/1 -> Id computation/2(Vdc), Unit Delay3/1
  Id computation/1(Id) -> Controlled Current Source2/1
  Mux2/1 -> Mux4/1  "Iabc"
  Mux4/1 -> Id computation/1(m)
  Current Measurement2/1 -> Mux2/3
  Mux/1 -> Mux4/2
  Voltage Measurement1/1 -> Mux/2  "Vbc"
  Voltage Measurement/1 -> Mux/1  "Vac"
  Current Measurement1/1 -> Mux2/2
  Current Measurement/1 -> Mux2/1
  connections:
  Activation Switches/LConn3 -- Controlled Voltage Source1/LConn1
  Controlled Voltage Source/RConn1 -- Activation Switches/LConn1
  C/RConn1 -- Current Measurement2/RConn1
  Current Measurement1/RConn1 -- B/RConn1
  Current Measurement/RConn1 -- A/RConn1
  Current Measurement1/LConn1 -- Activation Switches/RConn2 -- Voltage Measurement1/LConn1
  Controlled Voltage Source1/RConn1 -- Activation Switches/LConn2 -- Controlled Voltage Source/LConn1
  Current Measurement2/LConn1 -- Voltage Measurement1/LConn2 -- Activation Switches/RConn3 -- Voltage Measurement/LConn2
  Controlled Current Source1/RConn1 -- Activation Switches/LConn5 -- Output Resistance/LConn2
  Controlled Current Source/RConn1 -- Activation Switches/LConn4 -- Output Resistance/LConn1
  Current Measurement/LConn1 -- Activation Switches/RConn1 -- Voltage Measurement/LConn1
  Output Resistance/RConn1 -- Output Resistance/RConn2 -- Output Resistance/RConn3
  Output Resistance/LConn3 -- Controlled Current Source1/LConn1 -- Controlled Current Source/LConn1 -- Activation Switches/LConn6
  -/RConn1 -- Controlled Current Source2/RConn1 -- Voltage Measurement3/LConn2
  +/RConn1 -- Controlled Current Source2/LConn1 -- Voltage Measurement3/LConn1

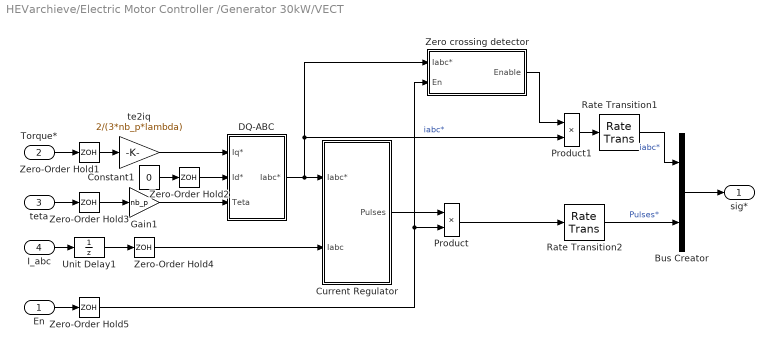
== system HEVarchieve/Electric Motor Controller /Generator 30kW/VECT ==
  En : Inport
  Torque* : Inport  Port=2
  teta : Inport  Port=3
  I_abc : Inport  Port=4
  Bus Creator : BusCreator  Inputs=2
  Constant1 : Constant  Value=0
  Current Regulator : Subsystem
  DQ-ABC : Subsystem
  Gain1 : Gain  Gain=nb_p  SaturateOnIntegerOverflow=on  OutDataTypeStr=Inherit: Same as input  ParamDataTypeStr=Inherit: Same as input
  Product : Product  RndMeth=Zero
  Product1 : Product  RndMeth=Zero
  Rate Transition1 : RateTransition
  Rate Transition2 : RateTransition
  Unit Delay1 : UnitDelay  SampleTime=Ts
  Zero crossing detector : Subsystem
  Zero-Order Hold{1..5} (5 alike) : ZeroOrderHold  SampleTime=Ts_vect
  te2iq : Gain  Gain=2/(3*nb_p*lambda)  SaturateOnIntegerOverflow=on  OutDataTypeStr=Inherit: Same as input  ParamDataTypeStr=Inherit: Same as input
  sig* : Outport
  wires:
  Zero-Order Hold5/1 -> Zero crossing detector/2(En), Product/2
  Zero crossing detector/1(Enable) -> Product1/1
  En/1 -> Zero-Order Hold5/1
  Product1/1 -> Rate Transition1/1
  Product/1 -> Rate Transition2/1
  Current Regulator/1(Pulses) -> Product/1
  Zero-Order Hold4/1 -> Current Regulator/2(Iabc)
  Rate Transition1/1 -> Bus Creator/1  "iabc*"
  Rate Transition2/1 -> Bus Creator/2  "Pulses*"
  Bus Creator/1 -> sig*/1
  te2iq/1 -> DQ-ABC/1("Iq* ")
  Zero-Order Hold2/1 -> DQ-ABC/2("Id* ")
  Zero-Order Hold1/1 -> te2iq/1
  teta/1 -> Zero-Order Hold3/1
  Zero-Order Hold3/1 -> Gain1/1
  Torque*/1 -> Zero-Order Hold1/1
  Constant1/1 -> Zero-Order Hold2/1
  Gain1/1 -> DQ-ABC/3(Teta)
  Unit Delay1/1 -> Zero-Order Hold4/1
  DQ-ABC/1(Iabc*) -> Zero crossing detector/1(Iabc*), Product1/2, Current Regulator/1(Iabc*)  "iabc*"
  I_abc/1 -> Unit Delay1/1

== system HEVarchieve/Electric Motor Controller /Motor 50kW/Mux ==
  sig : Inport
  m : Inport  Port=2
  Bus Creator : BusCreator  Inputs=2
  Ctrl : Outport
  wires:
  Bus Creator/1 -> Ctrl/1
  sig/1 -> Bus Creator/1  "sig"
  m/1 -> Bus Creator/2  "m"

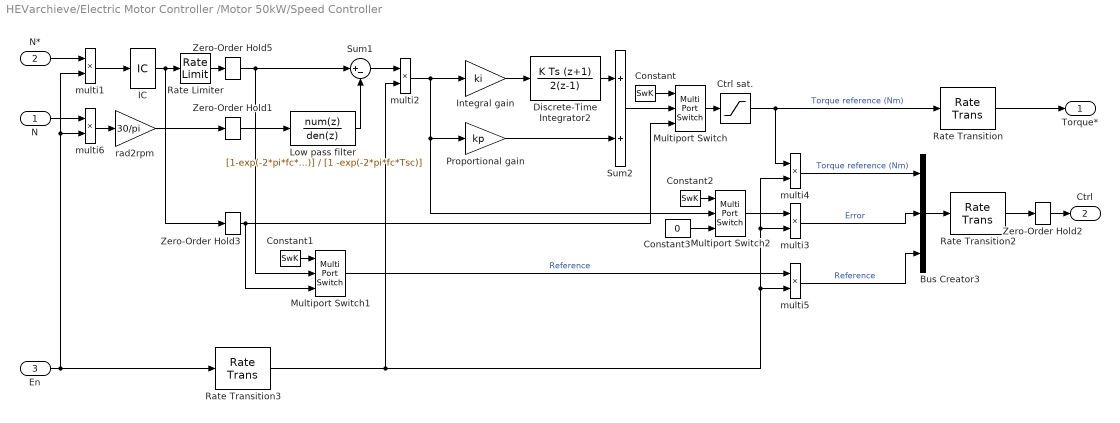
== system HEVarchieve/Electric Motor Controller /Motor 50kW/Speed Controller ==
  N : Inport
  N* : Inport  Port=2
  En : Inport  Port=3
  Bus Creator3 : BusCreator  Inputs=3
  Constant : Constant  Value=SwK
  Constant1 : Constant  Value=SwK
  Constant2 : Constant  Value=SwK
  Constant3 : Constant  Value=0
  Ctrl sat. : Saturate  UpperLimit=ctrl_sat(2)  LowerLimit=ctrl_sat(1)
  Discrete-Time Integrator2 : DiscreteIntegrator  IntegratorMethod=Integration: Trapezoidal  SampleTime=Tsc  LimitOutput=on  UpperSaturationLimit=ctrl_sat(2)  LowerSaturationLimit=ctrl_sat(1)
  IC : InitialCondition  Value=0
  Integral gain : Gain  Gain=ki  SaturateOnIntegerOverflow=on  OutDataTypeStr=Inherit: Same as input  ParamDataTypeStr=Inherit: Same as input
  Low pass filter : DiscreteTransferFcn  Numerator=[1-exp(-2*pi*fc*Tsc)]  Denominator=[1 -exp(-2*pi*fc*Tsc)]  SampleTime=Tsc
  Multiport Switch : MultiPortSwitch  Inputs=2  SaturateOnIntegerOverflow=on
  Multiport Switch1 : MultiPortSwitch  Inputs=2  SaturateOnIntegerOverflow=on
  Multiport Switch2 : MultiPortSwitch  Inputs=2  SaturateOnIntegerOverflow=on
  Proportional gain : Gain  Gain=kp  SaturateOnIntegerOverflow=on  OutDataTypeStr=Inherit: Same as input  ParamDataTypeStr=Inherit: Same as input
  Rate Limiter : RateLimiter  RisingSlewLimit=ramp(2)  FallingSlewLimit=ramp(1)  LinearizeAsGain=off
  Rate Transition : RateTransition
  Rate Transition2 : RateTransition
  Rate Transition3 : RateTransition
  Sum1 : Sum  Inputs=|+-  SaturateOnIntegerOverflow=on  InputSameDT=on  OutDataTypeStr=Inherit: Same as first input
  Sum2 : Sum  SaturateOnIntegerOverflow=on  InputSameDT=on  OutDataTypeStr=Inherit: Same as first input
  Zero-Order Hold1 : ZeroOrderHold  SampleTime=Tsc
  Zero-Order Hold2 : ZeroOrderHold  SampleTime=Ts
  Zero-Order Hold3 : ZeroOrderHold  SampleTime=Tsc
  Zero-Order Hold5 : ZeroOrderHold  SampleTime=Tsc
  multi{1..6} (6 alike) : Product
  rad2rpm : Gain  Gain=30/pi  SaturateOnIntegerOverflow=on  OutDataTypeStr=Inherit: Same as input  ParamDataTypeStr=Inherit: Same as input
  Torque* : Outport
  Ctrl : Outport  Port=2
  wires:
  Ctrl sat./1 -> multi4/1, Rate Transition/1  "Torque reference (Nm)"
  Integral gain/1 -> Discrete-Time Integrator2/1
  Sum1/1 -> multi2/1
  Discrete-Time Integrator2/1 -> Sum2/1
  Proportional gain/1 -> Sum2/2
  IC/1 -> Rate Limiter/1, Zero-Order Hold3/1
  Zero-Order Hold1/1 -> Low pass filter/1
  Rate Transition2/1 -> Zero-Order Hold2/1
  Bus Creator3/1 -> Rate Transition2/1
  Low pass filter/1 -> Sum1/2
  Rate Limiter/1 -> Zero-Order Hold5/1
  Zero-Order Hold5/1 -> Sum1/1, Multiport Switch1/2
  Multiport Switch/1 -> Ctrl sat./1
  Constant/1 -> Multiport Switch/1
  Sum2/1 -> Multiport Switch/2
  Constant1/1 -> Multiport Switch1/1
  Zero-Order Hold3/1 -> Multiport Switch/3, Multiport Switch1/3
  Constant2/1 -> Multiport Switch2/1
  Constant3/1 -> Multiport Switch2/3
  rad2rpm/1 -> Zero-Order Hold1/1
  En/1 -> Rate Transition3/1, multi1/2, multi6/2
  Rate Transition/1 -> Torque*/1
  Zero-Order Hold2/1 -> Ctrl/1
  Multiport Switch2/1 -> multi3/1
  multi3/1 -> Bus Creator3/2  "Error"
  multi5/1 -> Bus Creator3/3  "Reference"
  Multiport Switch1/1 -> multi5/1  "Reference"
  multi4/1 -> Bus Creator3/1  "Torque reference (Nm)"
  multi2/1 -> Integral gain/1, Proportional gain/1, Multiport Switch2/2
  Rate Transition3/1 -> multi2/2, multi4/2, multi3/2, multi5/2
  multi6/1 -> rad2rpm/1
  multi1/1 -> IC/1
  N*/1 -> multi1/1
  N/1 -> multi6/1

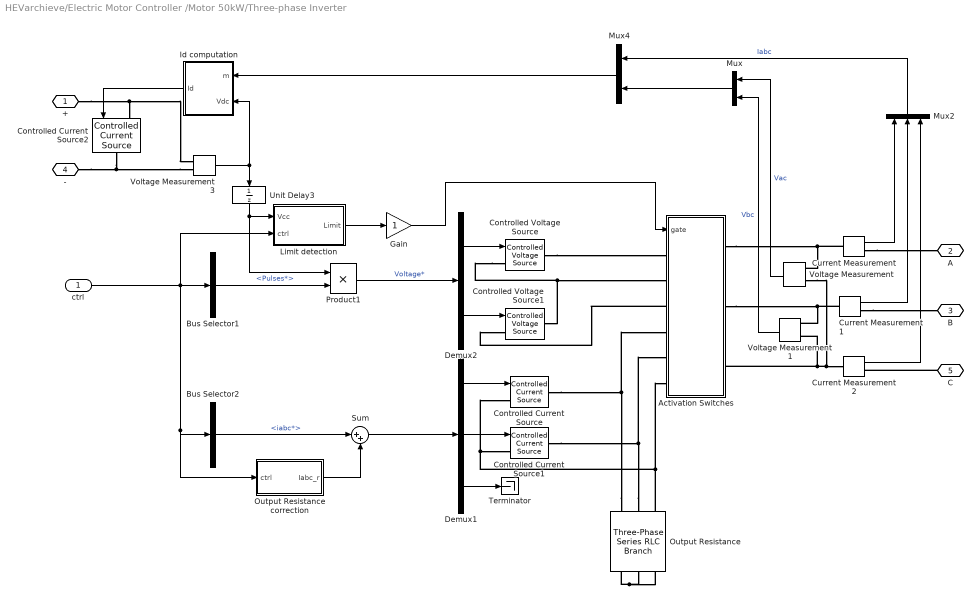
== system HEVarchieve/Electric Motor Controller /Motor 50kW/Three-phase Inverter ==
  ctrl : Inport
  Activation Switches : Subsystem
  Bus Selector1 : BusSelector  OutputSignals=sig.Pulses*
  Bus Selector2 : BusSelector  OutputSignals=sig.iabc*
  Controlled Current Source : powerlib/Electrical Sources/Controlled Current Source  Initialize=on  Source_Type=AC  Amplitude=0  Phase=0  Frequency=0  Measurements=None
  Controlled Current Source1 : powerlib/Electrical Sources/Controlled Current Source  Initialize=on  Source_Type=AC  Amplitude=0  Phase=0  Frequency=0  Measurements=None
  Controlled Current Source2 : powerlib/Electrical Sources/Controlled Current Source  Initialize=on  Source_Type=AC  Amplitude=0  Phase=0  Frequency=0  Measurements=None
  Controlled Voltage Source : powerlib/Electrical Sources/Controlled Voltage Source  Initialize=on  Source_Type=AC  Amplitude=0  Phase=0  Frequency=0  Measurements=None
  Controlled Voltage Source1 : powerlib/Electrical Sources/Controlled Voltage Source  Initialize=on  Source_Type=AC  Amplitude=0  Phase=0  Frequency=0  Measurements=None
  Current Measurement : powerlib/Measurements/Current Measurement  PhasorSimulation=off  OutputType=Complex  PSBequivalent=0
  Current Measurement1 : powerlib/Measurements/Current Measurement  PhasorSimulation=off  OutputType=Complex  PSBequivalent=0
  Current Measurement2 : powerlib/Measurements/Current Measurement  PhasorSimulation=off  OutputType=Complex  PSBequivalent=0
  Demux1 : Demux  Outputs=3
  Demux2 : Demux  Outputs=2
  Gain : Gain
  Id computation : Subsystem
  Limit detection : Subsystem
  Mux : Mux  Inputs=2
  Mux2 : Mux  Inputs=3
  Mux4 : Mux  Inputs=2
  Output Resistance : powerlib/Elements/Three-Phase Series RLC Branch  LConnTagsString=A|B|C  RConnTagsString=A|B|C  BranchType=R  Resistance=100*Resistance  Inductance=1e-3  Capacitance=1e-6  Measurements=Branch voltages and currents
  Output Resistance correction : Subsystem
  Product1 : Product  RndMeth=Zero
  Sum : Sum  Inputs=|++
  Terminator : Terminator
  Unit Delay3 : UnitDelay  SampleTime=Ts
  Voltage Measurement : powerlib/Measurements/Voltage Measurement  PhasorSimulation=off  OutputType=Complex  PSBequivalent=0
  Voltage Measurement1 : powerlib/Measurements/Voltage Measurement  PhasorSimulation=off  OutputType=Complex  PSBequivalent=0
  Voltage Measurement3 : powerlib/Measurements/Voltage Measurement  PhasorSimulation=off  OutputType=Complex  PSBequivalent=0
  + : PMIOPort  Port=1  Side=Right
  A : PMIOPort  Port=2  Side=Left
  B : PMIOPort  Port=3  Side=Left
  - : PMIOPort  Port=4  Side=Right
  C : PMIOPort  Port=5  Side=Left
  wires:
  Current Measurement/1 -> Mux2/1
  Current Measurement1/1 -> Mux2/2
  Voltage Measurement/1 -> Mux/1  "Vac"
  Voltage Measurement1/1 -> Mux/2  "Vbc"
  Mux/1 -> Mux4/2
  Current Measurement2/1 -> Mux2/3
  Mux4/1 -> Id computation/1(m)
  Mux2/1 -> Mux4/1  "Iabc"
  Voltage Measurement3/1 -> Unit Delay3/1, Id computation/2(Vdc)
  Bus Selector1/1 -> Product1/2  "<Pulses*>"
  Demux1/1 -> Controlled Current Source/1
  Demux1/2 -> Controlled Current Source1/1
  Demux1/3 -> Terminator/1
  Demux2/2 -> Controlled Voltage Source1/1
  Demux2/1 -> Controlled Voltage Source/1
  Bus Selector2/1 -> Sum/1  "<iabc*>"
  Limit detection/1(Limit) -> Gain/1
  Sum/1 -> Demux1/1
  Unit Delay3/1 -> Product1/1, Limit detection/1(Vcc)
  ctrl/1 -> Bus Selector1/1, Limit detection/2(ctrl), Bus Selector2/1, Output Resistance correction/1(ctrl)
  Product1/1 -> Demux2/1  "Voltage*"
  Gain/1 -> Activation Switches/1(gate)
  Id computation/1(Id) -> Controlled Current Source2/1
  Output Resistance correction/1("Iabc_r ") -> Sum/2
  connections:
  Voltage Measurement3/LConn1 -- Controlled Current Source2/LConn1 -- +/RConn1
  Voltage Measurement3/LConn2 -- Controlled Current Source2/RConn1 -- -/RConn1
  Activation Switches/LConn6 -- Controlled Current Source/LConn1 -- Controlled Current Source1/LConn1 -- Output Resistance/LConn3
  Output Resistance/RConn3 -- Output Resistance/RConn2 -- Output Resistance/RConn1
  Voltage Measurement/LConn1 -- Activation Switches/RConn1 -- Current Measurement/LConn1
  Output Resistance/LConn1 -- Activation Switches/LConn4 -- Controlled Current Source/RConn1
  Output Resistance/LConn2 -- Activation Switches/LConn5 -- Controlled Current Source1/RConn1
  Voltage Measurement/LConn2 -- Activation Switches/RConn3 -- Voltage Measurement1/LConn2 -- Current Measurement2/LConn1
  Controlled Voltage Source/LConn1 -- Activation Switches/LConn2 -- Controlled Voltage Source1/RConn1
  Voltage Measurement1/LConn1 -- Activation Switches/RConn2 -- Current Measurement1/LConn1
  Current Measurement/RConn1 -- A/RConn1
  Current Measurement1/RConn1 -- B/RConn1
  C/RConn1 -- Current Measurement2/RConn1
  Controlled Voltage Source/RConn1 -- Activation Switches/LConn1
  Activation Switches/LConn3 -- Controlled Voltage Source1/LConn1

== system HEVarchieve/Electric Motor Controller /Motor 50kW/Torque limitation ==
  N rad/s : Inport
  Torque : Inport  Port=2
  Abs1 : Abs  SaturateOnIntegerOverflow=on
  Gain : Gain  Gain=-1
  Saturation Dynamic : simulink/Discontinuities/Saturation Dynamic  OutMin=[]  OutMax=[]  OutDataTypeStr=Inherit: Same as second input  OutDataType=sfix(16)  OutScaling=2^-10  DoSatur=off
  Torque vs speed profile : Lookup  InputValues=[0 1200 2000 3000 4000 5000 6000]*pi/30  Table=[400 400 225 150 100 80 70]  LookUpMeth=Interpolation-Use End Values
  torque : Outport
  wires:
  N rad/s/1 -> Abs1/1
  Abs1/1 -> Torque vs speed profile/1
  Torque vs speed profile/1 -> Saturation Dynamic/1, Gain/1
  Saturation Dynamic/1 -> torque/1
  Torque/1 -> Saturation Dynamic/2
  Gain/1 -> Saturation Dynamic/3
